simulink model "approx_adders"  (R2021a)
settings: Solver=VariableStepAuto  StartTime=0.0  StopTime=10.0  RelTol=1e-3
libraries: xbsIndex_r4 x929
(part 2 of 2)

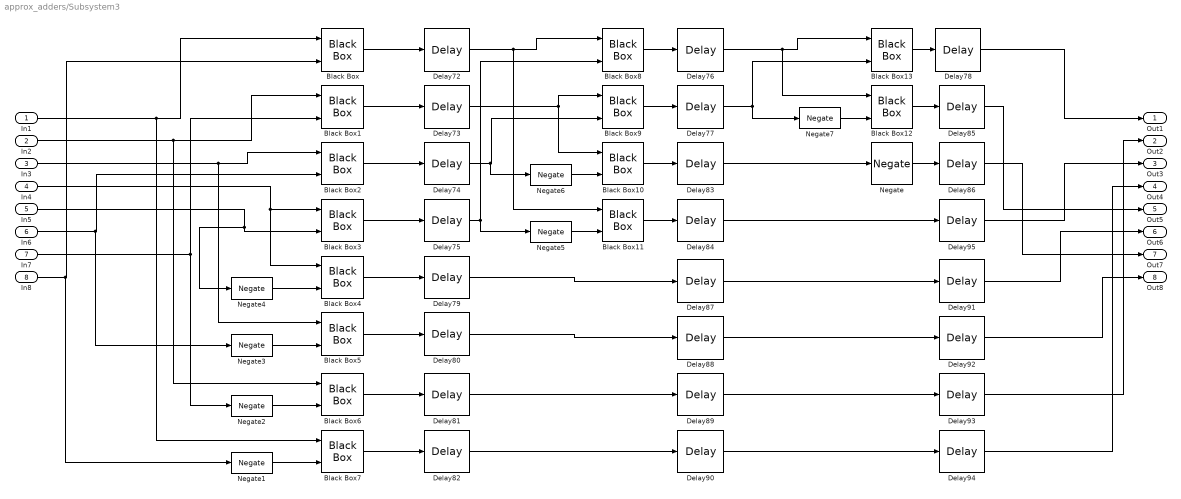
== system approx_adders/Subsystem3 ==
  In1 : Inport
  In2 : Inport  Port=2
  In3 : Inport  Port=3
  In4 : Inport  Port=4
  In5 : Inport  Port=5
  In6 : Inport  Port=6
  In7 : Inport  Port=7
  In8 : Inport  Port=8
  Black Box{,1..13} (14 alike) : xbsIndex_r4/Black Box  init_code=AA6_Multibit_config  sim_method=ISE Simulator  verbose=off  block_type=blackbox2
  Delay{72..95} (24 alike) : xbsIndex_r4/Delay  rst=off  infoeditControl=Selection of Reset will increase slice count due to use of real FFs and instead of SRLs  en=off  latency=1  reg_retiming=off  dbl_ovrd=off  block_type=delay
  Negate{,1..7} (8 alike) : xbsIndex_r4/Negate  precision=User Defined  arith_type="Signed  (2's comp)"  n_bits=Wa  bin_pt=Da  quantization="Round  (unbiased: +/- Inf)"  overflow=Saturate  en=off  latency=0  dbl_ovrd=off  block_type=negate
  Out1 : Outport
  Out2 : Outport  Port=2
  Out3 : Outport  Port=3
  Out4 : Outport  Port=4
  Out5 : Outport  Port=5
  Out6 : Outport  Port=6
  Out7 : Outport  Port=7
  Out8 : Outport  Port=8
  wires:
  Delay86/1 -> Out7/1
  Negate/1 -> Delay86/1
  Delay90/1 -> Delay94/1
  Delay84/1 -> Delay95/1
  Delay88/1 -> Delay92/1
  Delay92/1 -> Out8/1
  Delay87/1 -> Delay91/1
  Delay83/1 -> Negate/1
  Delay82/1 -> Delay90/1
  Delay91/1 -> Out6/1
  Delay80/1 -> Delay88/1
  Delay81/1 -> Delay89/1
  Delay78/1 -> Out1/1
  Delay79/1 -> Delay87/1
  Delay89/1 -> Delay93/1
  Delay95/1 -> Out3/1
  Delay94/1 -> Out4/1
  Delay85/1 -> Out5/1
  Delay93/1 -> Out2/1
  Black Box/1 -> Delay72/1
  Black Box1/1 -> Delay73/1
  Black Box2/1 -> Delay74/1
  Black Box3/1 -> Delay75/1
  Black Box4/1 -> Delay79/1
  Black Box5/1 -> Delay80/1
  Black Box6/1 -> Delay81/1
  Black Box7/1 -> Delay82/1
  Black Box8/1 -> Delay76/1
  Black Box9/1 -> Delay77/1
  Black Box10/1 -> Delay83/1
  Black Box11/1 -> Delay84/1
  Negate5/1 -> Black Box11/2
  Negate6/1 -> Black Box10/2
  Negate7/1 -> Black Box12/2
  Negate4/1 -> Black Box4/2
  Negate3/1 -> Black Box5/2
  Negate2/1 -> Black Box6/2
  Negate1/1 -> Black Box7/2
  Black Box13/1 -> Delay78/1
  Black Box12/1 -> Delay85/1
  Delay76/1 -> Black Box12/1, Black Box13/1
  Delay77/1 -> Black Box13/2, Negate7/1
  Delay72/1 -> Black Box11/1, Black Box8/1
  Delay73/1 -> Black Box9/1, Black Box10/1
  Delay74/1 -> Negate6/1, Black Box9/2
  Delay75/1 -> Negate5/1, Black Box8/2
  In1/1 -> Black Box7/1, Black Box/1
  In2/1 -> Black Box6/1, Black Box1/1
  In3/1 -> Black Box5/1, Black Box2/1
  In4/1 -> Black Box4/1, Black Box3/1
  In5/1 -> Negate4/1, Black Box3/2
  In6/1 -> Negate3/1, Black Box2/2
  In7/1 -> Black Box1/2, Negate2/1
  In8/1 -> Negate1/1, Black Box/2

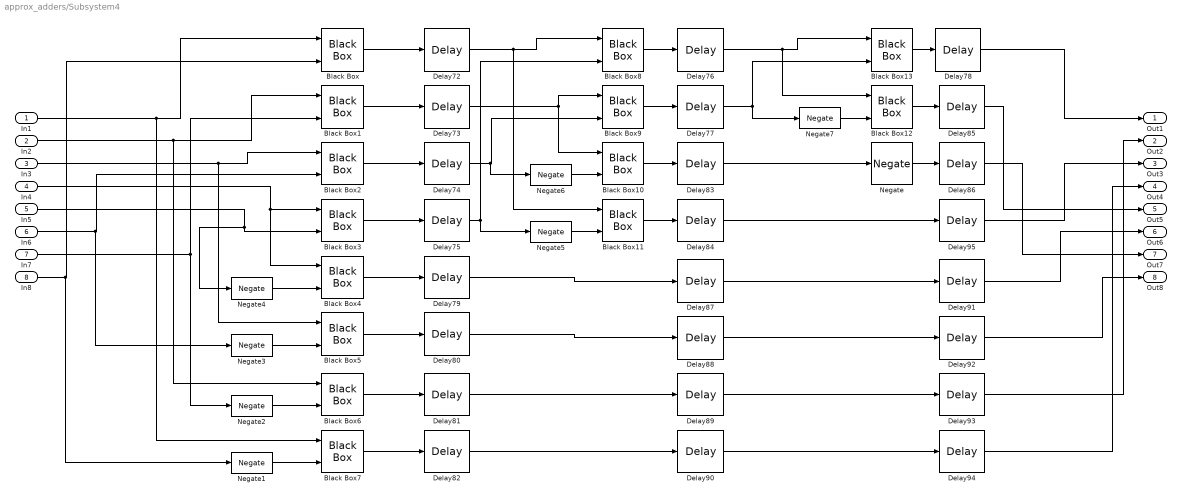
== system approx_adders/Subsystem4 ==
  In1 : Inport
  In2 : Inport  Port=2
  In3 : Inport  Port=3
  In4 : Inport  Port=4
  In5 : Inport  Port=5
  In6 : Inport  Port=6
  In7 : Inport  Port=7
  In8 : Inport  Port=8
  Black Box{,1..13} (14 alike) : xbsIndex_r4/Black Box  init_code=AA6_Multibit_config  sim_method=ISE Simulator  verbose=off  block_type=blackbox2
  Delay{72..95} (24 alike) : xbsIndex_r4/Delay  rst=off  infoeditControl=Selection of Reset will increase slice count due to use of real FFs and instead of SRLs  en=off  latency=1  reg_retiming=off  dbl_ovrd=off  block_type=delay
  Negate{,1..7} (8 alike) : xbsIndex_r4/Negate  precision=User Defined  arith_type="Signed  (2's comp)"  n_bits=Wa  bin_pt=Da  quantization="Round  (unbiased: +/- Inf)"  overflow=Saturate  en=off  latency=0  dbl_ovrd=off  block_type=negate
  Out1 : Outport
  Out2 : Outport  Port=2
  Out3 : Outport  Port=3
  Out4 : Outport  Port=4
  Out5 : Outport  Port=5
  Out6 : Outport  Port=6
  Out7 : Outport  Port=7
  Out8 : Outport  Port=8
  wires:
  Delay86/1 -> Out7/1
  Negate/1 -> Delay86/1
  Delay90/1 -> Delay94/1
  Delay84/1 -> Delay95/1
  Delay88/1 -> Delay92/1
  Delay92/1 -> Out8/1
  Delay87/1 -> Delay91/1
  Delay83/1 -> Negate/1
  Delay82/1 -> Delay90/1
  Delay91/1 -> Out6/1
  Delay80/1 -> Delay88/1
  Delay81/1 -> Delay89/1
  Delay78/1 -> Out1/1
  Delay79/1 -> Delay87/1
  Delay89/1 -> Delay93/1
  Delay95/1 -> Out3/1
  Delay94/1 -> Out4/1
  Delay85/1 -> Out5/1
  Delay93/1 -> Out2/1
  Black Box/1 -> Delay72/1
  Black Box1/1 -> Delay73/1
  Black Box2/1 -> Delay74/1
  Black Box3/1 -> Delay75/1
  Black Box4/1 -> Delay79/1
  Black Box5/1 -> Delay80/1
  Black Box6/1 -> Delay81/1
  Black Box7/1 -> Delay82/1
  Black Box8/1 -> Delay76/1
  Black Box9/1 -> Delay77/1
  Black Box10/1 -> Delay83/1
  Black Box11/1 -> Delay84/1
  Negate5/1 -> Black Box11/2
  Negate6/1 -> Black Box10/2
  Negate7/1 -> Black Box12/2
  Negate4/1 -> Black Box4/2
  Negate3/1 -> Black Box5/2
  Negate2/1 -> Black Box6/2
  Negate1/1 -> Black Box7/2
  Black Box13/1 -> Delay78/1
  Black Box12/1 -> Delay85/1
  Delay76/1 -> Black Box12/1, Black Box13/1
  Delay77/1 -> Black Box13/2, Negate7/1
  Delay72/1 -> Black Box11/1, Black Box8/1
  Delay73/1 -> Black Box9/1, Black Box10/1
  Delay74/1 -> Negate6/1, Black Box9/2
  Delay75/1 -> Negate5/1, Black Box8/2
  In1/1 -> Black Box7/1, Black Box/1
  In2/1 -> Black Box6/1, Black Box1/1
  In3/1 -> Black Box5/1, Black Box2/1
  In4/1 -> Black Box4/1, Black Box3/1
  In5/1 -> Negate4/1, Black Box3/2
  In6/1 -> Negate3/1, Black Box2/2
  In7/1 -> Black Box1/2, Negate2/1
  In8/1 -> Negate1/1, Black Box/2

== system approx_adders/Subsystem5 ==
  In1 : Inport
  In2 : Inport  Port=2
  In3 : Inport  Port=3
  In4 : Inport  Port=4
  In5 : Inport  Port=5
  In6 : Inport  Port=6
  In7 : Inport  Port=7
  In8 : Inport  Port=8
  Black Box{,1..13} (14 alike) : xbsIndex_r4/Black Box  init_code=AA6_Multibit_config  sim_method=ISE Simulator  verbose=off  block_type=blackbox2
  Delay{72..95} (24 alike) : xbsIndex_r4/Delay  rst=off  infoeditControl=Selection of Reset will increase slice count due to use of real FFs and instead of SRLs  en=off  latency=1  reg_retiming=off  dbl_ovrd=off  block_type=delay
  Negate{,1..7} (8 alike) : xbsIndex_r4/Negate  precision=User Defined  arith_type="Signed  (2's comp)"  n_bits=Wa  bin_pt=Da  quantization="Round  (unbiased: +/- Inf)"  overflow=Saturate  en=off  latency=0  dbl_ovrd=off  block_type=negate
  Out1 : Outport
  Out2 : Outport  Port=2
  Out3 : Outport  Port=3
  Out4 : Outport  Port=4
  Out5 : Outport  Port=5
  Out6 : Outport  Port=6
  Out7 : Outport  Port=7
  Out8 : Outport  Port=8
  wires:
  Delay86/1 -> Out7/1
  Negate/1 -> Delay86/1
  Delay90/1 -> Delay94/1
  Delay84/1 -> Delay95/1
  Delay88/1 -> Delay92/1
  Delay92/1 -> Out8/1
  Delay87/1 -> Delay91/1
  Delay83/1 -> Negate/1
  Delay82/1 -> Delay90/1
  Delay91/1 -> Out6/1
  Delay80/1 -> Delay88/1
  Delay81/1 -> Delay89/1
  Delay78/1 -> Out1/1
  Delay79/1 -> Delay87/1
  Delay89/1 -> Delay93/1
  Delay95/1 -> Out3/1
  Delay94/1 -> Out4/1
  Delay85/1 -> Out5/1
  Delay93/1 -> Out2/1
  Black Box/1 -> Delay72/1
  Black Box1/1 -> Delay73/1
  Black Box2/1 -> Delay74/1
  Black Box3/1 -> Delay75/1
  Black Box4/1 -> Delay79/1
  Black Box5/1 -> Delay80/1
  Black Box6/1 -> Delay81/1
  Black Box7/1 -> Delay82/1
  Black Box8/1 -> Delay76/1
  Black Box9/1 -> Delay77/1
  Black Box10/1 -> Delay83/1
  Black Box11/1 -> Delay84/1
  Negate5/1 -> Black Box11/2
  Negate6/1 -> Black Box10/2
  Negate7/1 -> Black Box12/2
  Negate4/1 -> Black Box4/2
  Negate3/1 -> Black Box5/2
  Negate2/1 -> Black Box6/2
  Negate1/1 -> Black Box7/2
  Black Box13/1 -> Delay78/1
  Black Box12/1 -> Delay85/1
  Delay76/1 -> Black Box12/1, Black Box13/1
  Delay77/1 -> Black Box13/2, Negate7/1
  Delay72/1 -> Black Box11/1, Black Box8/1
  Delay73/1 -> Black Box9/1, Black Box10/1
  Delay74/1 -> Negate6/1, Black Box9/2
  Delay75/1 -> Negate5/1, Black Box8/2
  In1/1 -> Black Box7/1, Black Box/1
  In2/1 -> Black Box6/1, Black Box1/1
  In3/1 -> Black Box5/1, Black Box2/1
  In4/1 -> Black Box4/1, Black Box3/1
  In5/1 -> Negate4/1, Black Box3/2
  In6/1 -> Negate3/1, Black Box2/2
  In7/1 -> Black Box1/2, Negate2/1
  In8/1 -> Negate1/1, Black Box/2

== system approx_adders/Subsystem6 ==
  In1 : Inport
  In2 : Inport  Port=2
  In3 : Inport  Port=3
  In4 : Inport  Port=4
  In5 : Inport  Port=5
  In6 : Inport  Port=6
  In7 : Inport  Port=7
  In8 : Inport  Port=8
  Black Box{,1..13} (14 alike) : xbsIndex_r4/Black Box  init_code=AA6_Multibit_config  sim_method=ISE Simulator  verbose=off  block_type=blackbox2
  Delay{72..95} (24 alike) : xbsIndex_r4/Delay  rst=off  infoeditControl=Selection of Reset will increase slice count due to use of real FFs and instead of SRLs  en=off  latency=1  reg_retiming=off  dbl_ovrd=off  block_type=delay
  Negate{,1..7} (8 alike) : xbsIndex_r4/Negate  precision=User Defined  arith_type="Signed  (2's comp)"  n_bits=Wa  bin_pt=Da  quantization="Round  (unbiased: +/- Inf)"  overflow=Saturate  en=off  latency=0  dbl_ovrd=off  block_type=negate
  Out1 : Outport
  Out2 : Outport  Port=2
  Out3 : Outport  Port=3
  Out4 : Outport  Port=4
  Out5 : Outport  Port=5
  Out6 : Outport  Port=6
  Out7 : Outport  Port=7
  Out8 : Outport  Port=8
  wires:
  Delay86/1 -> Out7/1
  Negate/1 -> Delay86/1
  Delay90/1 -> Delay94/1
  Delay84/1 -> Delay95/1
  Delay88/1 -> Delay92/1
  Delay92/1 -> Out8/1
  Delay87/1 -> Delay91/1
  Delay83/1 -> Negate/1
  Delay82/1 -> Delay90/1
  Delay91/1 -> Out6/1
  Delay80/1 -> Delay88/1
  Delay81/1 -> Delay89/1
  Delay78/1 -> Out1/1
  Delay79/1 -> Delay87/1
  Delay89/1 -> Delay93/1
  Delay95/1 -> Out3/1
  Delay94/1 -> Out4/1
  Delay85/1 -> Out5/1
  Delay93/1 -> Out2/1
  Black Box/1 -> Delay72/1
  Black Box1/1 -> Delay73/1
  Black Box2/1 -> Delay74/1
  Black Box3/1 -> Delay75/1
  Black Box4/1 -> Delay79/1
  Black Box5/1 -> Delay80/1
  Black Box6/1 -> Delay81/1
  Black Box7/1 -> Delay82/1
  Black Box8/1 -> Delay76/1
  Black Box9/1 -> Delay77/1
  Black Box10/1 -> Delay83/1
  Black Box11/1 -> Delay84/1
  Negate5/1 -> Black Box11/2
  Negate6/1 -> Black Box10/2
  Negate7/1 -> Black Box12/2
  Negate4/1 -> Black Box4/2
  Negate3/1 -> Black Box5/2
  Negate2/1 -> Black Box6/2
  Negate1/1 -> Black Box7/2
  Black Box13/1 -> Delay78/1
  Black Box12/1 -> Delay85/1
  Delay76/1 -> Black Box12/1, Black Box13/1
  Delay77/1 -> Black Box13/2, Negate7/1
  Delay72/1 -> Black Box11/1, Black Box8/1
  Delay73/1 -> Black Box9/1, Black Box10/1
  Delay74/1 -> Negate6/1, Black Box9/2
  Delay75/1 -> Negate5/1, Black Box8/2
  In1/1 -> Black Box7/1, Black Box/1
  In2/1 -> Black Box6/1, Black Box1/1
  In3/1 -> Black Box5/1, Black Box2/1
  In4/1 -> Black Box4/1, Black Box3/1
  In5/1 -> Negate4/1, Black Box3/2
  In6/1 -> Negate3/1, Black Box2/2
  In7/1 -> Black Box1/2, Negate2/1
  In8/1 -> Negate1/1, Black Box/2

== system approx_adders/Subsystem7 ==
  In1 : Inport
  In2 : Inport  Port=2
  In3 : Inport  Port=3
  In4 : Inport  Port=4
  In5 : Inport  Port=5
  In6 : Inport  Port=6
  In7 : Inport  Port=7
  In8 : Inport  Port=8
  Black Box{,1..13} (14 alike) : xbsIndex_r4/Black Box  init_code=AA6_Multibit_config  sim_method=ISE Simulator  verbose=off  block_type=blackbox2
  Delay{72..95} (24 alike) : xbsIndex_r4/Delay  rst=off  infoeditControl=Selection of Reset will increase slice count due to use of real FFs and instead of SRLs  en=off  latency=1  reg_retiming=off  dbl_ovrd=off  block_type=delay
  Negate{,1..7} (8 alike) : xbsIndex_r4/Negate  precision=User Defined  arith_type="Signed  (2's comp)"  n_bits=Wa  bin_pt=Da  quantization="Round  (unbiased: +/- Inf)"  overflow=Saturate  en=off  latency=0  dbl_ovrd=off  block_type=negate
  Out1 : Outport
  Out2 : Outport  Port=2
  Out3 : Outport  Port=3
  Out4 : Outport  Port=4
  Out5 : Outport  Port=5
  Out6 : Outport  Port=6
  Out7 : Outport  Port=7
  Out8 : Outport  Port=8
  wires:
  Delay86/1 -> Out7/1
  Negate/1 -> Delay86/1
  Delay90/1 -> Delay94/1
  Delay84/1 -> Delay95/1
  Delay88/1 -> Delay92/1
  Delay92/1 -> Out8/1
  Delay87/1 -> Delay91/1
  Delay83/1 -> Negate/1
  Delay82/1 -> Delay90/1
  Delay91/1 -> Out6/1
  Delay80/1 -> Delay88/1
  Delay81/1 -> Delay89/1
  Delay78/1 -> Out1/1
  Delay79/1 -> Delay87/1
  Delay89/1 -> Delay93/1
  Delay95/1 -> Out3/1
  Delay94/1 -> Out4/1
  Delay85/1 -> Out5/1
  Delay93/1 -> Out2/1
  Black Box/1 -> Delay72/1
  Black Box1/1 -> Delay73/1
  Black Box2/1 -> Delay74/1
  Black Box3/1 -> Delay75/1
  Black Box4/1 -> Delay79/1
  Black Box5/1 -> Delay80/1
  Black Box6/1 -> Delay81/1
  Black Box7/1 -> Delay82/1
  Black Box8/1 -> Delay76/1
  Black Box9/1 -> Delay77/1
  Black Box10/1 -> Delay83/1
  Black Box11/1 -> Delay84/1
  Negate5/1 -> Black Box11/2
  Negate6/1 -> Black Box10/2
  Negate7/1 -> Black Box12/2
  Negate4/1 -> Black Box4/2
  Negate3/1 -> Black Box5/2
  Negate2/1 -> Black Box6/2
  Negate1/1 -> Black Box7/2
  Black Box13/1 -> Delay78/1
  Black Box12/1 -> Delay85/1
  Delay76/1 -> Black Box12/1, Black Box13/1
  Delay77/1 -> Black Box13/2, Negate7/1
  Delay72/1 -> Black Box11/1, Black Box8/1
  Delay73/1 -> Black Box9/1, Black Box10/1
  Delay74/1 -> Negate6/1, Black Box9/2
  Delay75/1 -> Negate5/1, Black Box8/2
  In1/1 -> Black Box7/1, Black Box/1
  In2/1 -> Black Box6/1, Black Box1/1
  In3/1 -> Black Box5/1, Black Box2/1
  In4/1 -> Black Box4/1, Black Box3/1
  In5/1 -> Negate4/1, Black Box3/2
  In6/1 -> Negate3/1, Black Box2/2
  In7/1 -> Black Box1/2, Negate2/1
  In8/1 -> Negate1/1, Black Box/2

== system approx_adders/Subsystem8 ==
  In1 : Inport
  In2 : Inport  Port=2
  In3 : Inport  Port=3
  In4 : Inport  Port=4
  In5 : Inport  Port=5
  In6 : Inport  Port=6
  In7 : Inport  Port=7
  In8 : Inport  Port=8
  Black Box{,1..13} (14 alike) : xbsIndex_r4/Black Box  init_code=AA6_Multibit_config  sim_method=ISE Simulator  verbose=off  block_type=blackbox2
  Delay{72..95} (24 alike) : xbsIndex_r4/Delay  rst=off  infoeditControl=Selection of Reset will increase slice count due to use of real FFs and instead of SRLs  en=off  latency=1  reg_retiming=off  dbl_ovrd=off  block_type=delay
  Negate{,1..7} (8 alike) : xbsIndex_r4/Negate  precision=User Defined  arith_type="Signed  (2's comp)"  n_bits=Wa  bin_pt=Da  quantization="Round  (unbiased: +/- Inf)"  overflow=Saturate  en=off  latency=0  dbl_ovrd=off  block_type=negate
  Out1 : Outport
  Out2 : Outport  Port=2
  Out3 : Outport  Port=3
  Out4 : Outport  Port=4
  Out5 : Outport  Port=5
  Out6 : Outport  Port=6
  Out7 : Outport  Port=7
  Out8 : Outport  Port=8
  wires:
  Delay86/1 -> Out7/1
  Negate/1 -> Delay86/1
  Delay90/1 -> Delay94/1
  Delay84/1 -> Delay95/1
  Delay88/1 -> Delay92/1
  Delay92/1 -> Out8/1
  Delay87/1 -> Delay91/1
  Delay83/1 -> Negate/1
  Delay82/1 -> Delay90/1
  Delay91/1 -> Out6/1
  Delay80/1 -> Delay88/1
  Delay81/1 -> Delay89/1
  Delay78/1 -> Out1/1
  Delay79/1 -> Delay87/1
  Delay89/1 -> Delay93/1
  Delay95/1 -> Out3/1
  Delay94/1 -> Out4/1
  Delay85/1 -> Out5/1
  Delay93/1 -> Out2/1
  Black Box/1 -> Delay72/1
  Black Box1/1 -> Delay73/1
  Black Box2/1 -> Delay74/1
  Black Box3/1 -> Delay75/1
  Black Box4/1 -> Delay79/1
  Black Box5/1 -> Delay80/1
  Black Box6/1 -> Delay81/1
  Black Box7/1 -> Delay82/1
  Black Box8/1 -> Delay76/1
  Black Box9/1 -> Delay77/1
  Black Box10/1 -> Delay83/1
  Black Box11/1 -> Delay84/1
  Negate5/1 -> Black Box11/2
  Negate6/1 -> Black Box10/2
  Negate7/1 -> Black Box12/2
  Negate4/1 -> Black Box4/2
  Negate3/1 -> Black Box5/2
  Negate2/1 -> Black Box6/2
  Negate1/1 -> Black Box7/2
  Black Box13/1 -> Delay78/1
  Black Box12/1 -> Delay85/1
  Delay76/1 -> Black Box12/1, Black Box13/1
  Delay77/1 -> Black Box13/2, Negate7/1
  Delay72/1 -> Black Box11/1, Black Box8/1
  Delay73/1 -> Black Box9/1, Black Box10/1
  Delay74/1 -> Negate6/1, Black Box9/2
  Delay75/1 -> Negate5/1, Black Box8/2
  In1/1 -> Black Box7/1, Black Box/1
  In2/1 -> Black Box6/1, Black Box1/1
  In3/1 -> Black Box5/1, Black Box2/1
  In4/1 -> Black Box4/1, Black Box3/1
  In5/1 -> Negate4/1, Black Box3/2
  In6/1 -> Negate3/1, Black Box2/2
  In7/1 -> Black Box1/2, Negate2/1
  In8/1 -> Negate1/1, Black Box/2

== system approx_adders/Subsystem9 ==
  In1 : Inport
  In2 : Inport  Port=2
  In3 : Inport  Port=3
  In4 : Inport  Port=4
  In5 : Inport  Port=5
  In6 : Inport  Port=6
  In7 : Inport  Port=7
  In8 : Inport  Port=8
  Black Box{,1..13} (14 alike) : xbsIndex_r4/Black Box  init_code=AA6_Multibit_config  sim_method=ISE Simulator  verbose=off  block_type=blackbox2
  Delay{72..95} (24 alike) : xbsIndex_r4/Delay  rst=off  infoeditControl=Selection of Reset will increase slice count due to use of real FFs and instead of SRLs  en=off  latency=1  reg_retiming=off  dbl_ovrd=off  block_type=delay
  Negate{,1..7} (8 alike) : xbsIndex_r4/Negate  precision=User Defined  arith_type="Signed  (2's comp)"  n_bits=Wa  bin_pt=Da  quantization="Round  (unbiased: +/- Inf)"  overflow=Saturate  en=off  latency=0  dbl_ovrd=off  block_type=negate
  Out1 : Outport
  Out2 : Outport  Port=2
  Out3 : Outport  Port=3
  Out4 : Outport  Port=4
  Out5 : Outport  Port=5
  Out6 : Outport  Port=6
  Out7 : Outport  Port=7
  Out8 : Outport  Port=8
  wires:
  Delay86/1 -> Out7/1
  Negate/1 -> Delay86/1
  Delay90/1 -> Delay94/1
  Delay84/1 -> Delay95/1
  Delay88/1 -> Delay92/1
  Delay92/1 -> Out8/1
  Delay87/1 -> Delay91/1
  Delay83/1 -> Negate/1
  Delay82/1 -> Delay90/1
  Delay91/1 -> Out6/1
  Delay80/1 -> Delay88/1
  Delay81/1 -> Delay89/1
  Delay78/1 -> Out1/1
  Delay79/1 -> Delay87/1
  Delay89/1 -> Delay93/1
  Delay95/1 -> Out3/1
  Delay94/1 -> Out4/1
  Delay85/1 -> Out5/1
  Delay93/1 -> Out2/1
  Black Box/1 -> Delay72/1
  Black Box1/1 -> Delay73/1
  Black Box2/1 -> Delay74/1
  Black Box3/1 -> Delay75/1
  Black Box4/1 -> Delay79/1
  Black Box5/1 -> Delay80/1
  Black Box6/1 -> Delay81/1
  Black Box7/1 -> Delay82/1
  Black Box8/1 -> Delay76/1
  Black Box9/1 -> Delay77/1
  Black Box10/1 -> Delay83/1
  Black Box11/1 -> Delay84/1
  Negate5/1 -> Black Box11/2
  Negate6/1 -> Black Box10/2
  Negate7/1 -> Black Box12/2
  Negate4/1 -> Black Box4/2
  Negate3/1 -> Black Box5/2
  Negate2/1 -> Black Box6/2
  Negate1/1 -> Black Box7/2
  Black Box13/1 -> Delay78/1
  Black Box12/1 -> Delay85/1
  Delay76/1 -> Black Box12/1, Black Box13/1
  Delay77/1 -> Black Box13/2, Negate7/1
  Delay72/1 -> Black Box11/1, Black Box8/1
  Delay73/1 -> Black Box9/1, Black Box10/1
  Delay74/1 -> Negate6/1, Black Box9/2
  Delay75/1 -> Negate5/1, Black Box8/2
  In1/1 -> Black Box7/1, Black Box/1
  In2/1 -> Black Box6/1, Black Box1/1
  In3/1 -> Black Box5/1, Black Box2/1
  In4/1 -> Black Box4/1, Black Box3/1
  In5/1 -> Negate4/1, Black Box3/2
  In6/1 -> Negate3/1, Black Box2/2
  In7/1 -> Black Box1/2, Negate2/1
  In8/1 -> Negate1/1, Black Box/2
